simulink model "HybridSystem"  (R2020a)
settings: Solver=FixedStepAuto  StartTime=0  StopTime=1000  FixedStep=0.01  RelTol=1e-3
undefined symbols (not defined in the file): K_I, K_P, n_delay, sac_thresh, switch_thresh, T_lim_low, T_lim_up
libraries: cstblocks x1, simulink x1
settings Model: Creator=Brock  LastModifiedBy=Brock

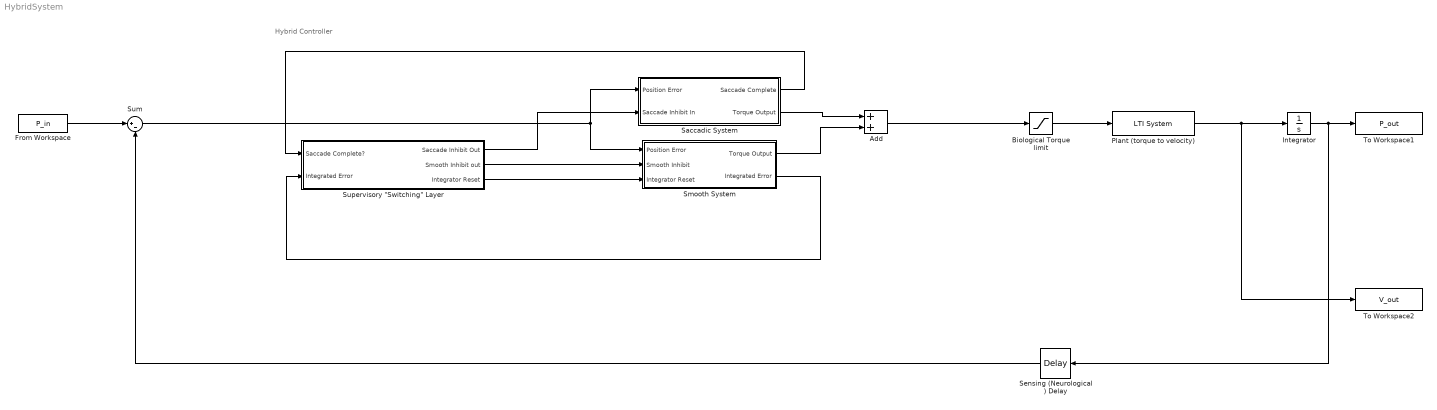
== system HybridSystem ==
  note: Hybrid Controller
  Add : Sum
  Biological Torque limit : Saturate  UpperLimit=T_lim_up  LowerLimit=T_lim_low  LinearizeAsGain=off
  From Workspace : FromWorkspace  VariableName=P_in
  Integrator : Integrator
  Plant (torque to velocity) : cstblocks/LTI System  sys=G_plant  IC=[]
  Saccadic System : Subsystem
  Sensing (Neurological) Delay : TransportDelay  DelayTime=n_delay
  Smooth System : Subsystem
  Sum : Sum  Inputs=|+-
  "Supervisory \"Switching\" Layer" : Subsystem
  To Workspace1 : ToWorkspace  VariableName=P_out  SampleTime=-1
  To Workspace2 : ToWorkspace  VariableName=V_out  SampleTime=-1
  wires:
  From Workspace/1 -> Sum/1
  Plant (torque to velocity)/1 -> Integrator/1, To Workspace2/1
  Integrator/1 -> Sensing (Neurological) Delay/1, To Workspace1/1
  Biological Torque limit/1 -> Plant (torque to velocity)/1
  Sensing (Neurological) Delay/1 -> Sum/2
  Add/1 -> Biological Torque limit/1
  Smooth System/1(Torque Output) -> Add/2
  Saccadic System/2(Torque Output) -> Add/1
  "Supervisory \"Switching\" Layer"/3(Integrator Reset) -> Smooth System/3(Integrator Reset)
  Smooth System/2(Integrated Error) -> "Supervisory \"Switching\" Layer"/2(Integrated Error)
  Sum/1 -> Saccadic System/1(Position Error), Smooth System/1(Position Error)
  Saccadic System/1(Saccade Complete) -> "Supervisory \"Switching\" Layer"/1(Saccade Complete?)
  "Supervisory \"Switching\" Layer"/2(Smooth Inhibit out) -> Smooth System/2(Smooth Inhibit)
  "Supervisory \"Switching\" Layer"/1(Saccade Inhibit Out) -> Saccadic System/2(Saccade Inhibit In)

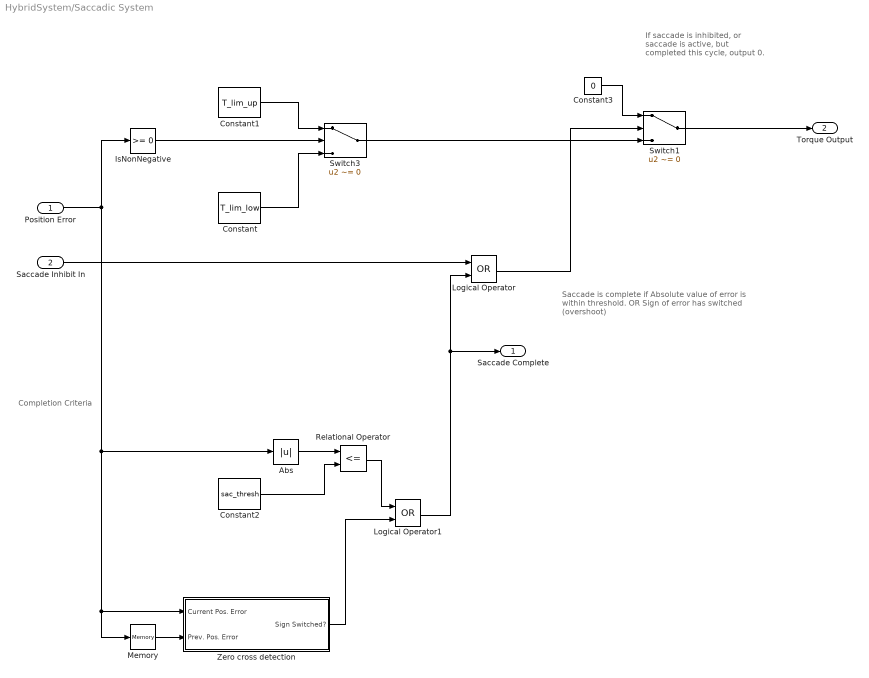
== system HybridSystem/Saccadic System ==
  note: Completion
      | Criteria
  note: If saccade is inhibited, or saccade is active, but completed this cycle, output 0.
  note: Saccade is complete if
      | Absolute value of error is within threshold.
      | OR
      | Sign of error has switched (overshoot)
  Position Error : Inport
  Saccade Inhibit In : Inport  Port=2
  Abs : Abs
  Constant : Constant  Value=T_lim_low
  Constant1 : Constant  Value=T_lim_up
  Constant2 : Constant  Value=sac_thresh
  Constant3 : Constant  Value=0
  IsNonNegative : simulink/Logic and Bit Operations/Compare To Zero  relop=>=  OutDataTypeStr=boolean
  Logical Operator : Logic  Operator=OR  AllPortsSameDT=off  OutDataTypeStr=boolean
  Logical Operator1 : Logic  Operator=OR  AllPortsSameDT=off  OutDataTypeStr=boolean
  Memory : Memory  InheritSampleTime=on
  Relational Operator : RelationalOperator  Operator=<=  OutDataTypeStr=boolean  RndMeth=Simplest
  Switch1 : Switch  Criteria=u2 ~= 0  Threshold=1
  Switch3 : Switch  Criteria=u2 ~= 0
  Zero cross detection : Subsystem
  Saccade Complete : Outport
  Torque Output : Outport  Port=2
  wires:
  Constant2/1 -> Relational Operator/2
  Position Error/1 -> Memory/1, Zero cross detection/1(Current Pos. Error), Abs/1, IsNonNegative/1
  Abs/1 -> Relational Operator/1
  Saccade Inhibit In/1 -> Logical Operator/1
  Switch1/1 -> Torque Output/1
  Constant3/1 -> Switch1/1
  Constant/1 -> Switch3/3
  Constant1/1 -> Switch3/1
  Logical Operator/1 -> Switch1/2
  Switch3/1 -> Switch1/3
  Relational Operator/1 -> Logical Operator1/1
  Logical Operator1/1 -> Logical Operator/2, Saccade Complete/1
  Zero cross detection/1(Sign Switched?) -> Logical Operator1/2
  IsNonNegative/1 -> Switch3/2
  Memory/1 -> Zero cross detection/2(Prev. Pos. Error)

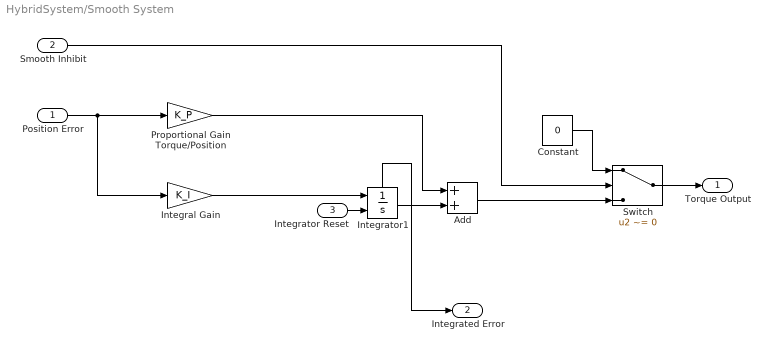
== system HybridSystem/Smooth System ==
  Position Error : Inport
  Smooth Inhibit : Inport  Port=2
  Integrator Reset : Inport  Port=3
  Add : Sum
  Constant : Constant  Value=0
  "Integral Gain " : Gain  Gain=K_I
  Integrator1 : Integrator  ExternalReset=rising  ShowStatePort=on
  Proportional Gain Torque/Position : Gain  Gain=K_P
  Switch : Switch  Criteria=u2 ~= 0
  Torque Output : Outport
  Integrated Error : Outport  Port=2
  wires:
  Proportional Gain Torque/Position/1 -> Add/1
  "Integral Gain "/1 -> Integrator1/1
  Integrator Reset/1 -> Integrator1/2
  Integrator1/1 -> Add/2
  Position Error/1 -> "Integral Gain "/1, Proportional Gain Torque/Position/1
  Switch/1 -> Torque Output/1
  Smooth Inhibit/1 -> Switch/2
  Add/1 -> Switch/3
  Constant/1 -> Switch/1
  Integrator1/State -> Integrated Error/1

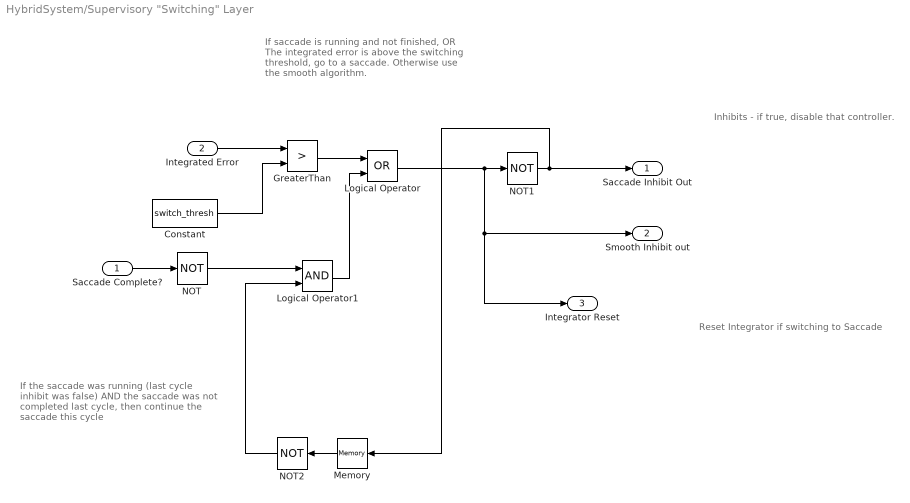
== system HybridSystem/Supervisory "Switching" Layer ==
  note: Inhibits - if true, disable that controller.
  note: If the saccade was running (last cycle inhibit was false)
      | AND the saccade was not completed last cycle, then continue
      | the saccade this cycle
  note: If saccade is running and not finished,
      | OR
      | The integrated error is above the switching threshold, go to a saccade.
      | Otherwise use the smooth algorithm.
  note: Reset Integrator if switching to Saccade
  Saccade Complete? : Inport
  Integrated Error : Inport  Port=2
  Constant : Constant  Value=switch_thresh
  GreaterThan : RelationalOperator  Operator=>  OutDataTypeStr=boolean  RndMeth=Simplest
  Logical Operator : Logic  Operator=OR  AllPortsSameDT=off  OutDataTypeStr=boolean
  Logical Operator1 : Logic  AllPortsSameDT=off  OutDataTypeStr=boolean
  Memory : Memory
  NOT : Logic  Operator=NOT  IconShape=distinctive  AllPortsSameDT=off  OutDataTypeStr=boolean
  NOT1 : Logic  Operator=NOT  IconShape=distinctive  AllPortsSameDT=off  OutDataTypeStr=boolean
  NOT2 : Logic  Operator=NOT  IconShape=distinctive  AllPortsSameDT=off  OutDataTypeStr=boolean
  Saccade Inhibit Out : Outport
  Smooth Inhibit out : Outport  Port=2
  Integrator Reset : Outport  Port=3
  wires:
  Integrated Error/1 -> GreaterThan/1
  Constant/1 -> GreaterThan/2
  Saccade Complete?/1 -> NOT/1
  GreaterThan/1 -> Logical Operator/1
  Logical Operator/1 -> NOT1/1, Smooth Inhibit out/1, Integrator Reset/1
  NOT1/1 -> Memory/1, Saccade Inhibit Out/1
  Logical Operator1/1 -> Logical Operator/2
  NOT/1 -> Logical Operator1/1
  Memory/1 -> NOT2/1
  NOT2/1 -> Logical Operator1/2

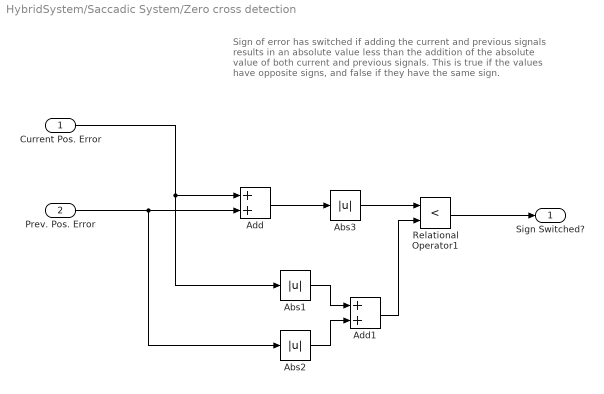
== system HybridSystem/Saccadic System/Zero cross detection ==
  note: Sign of error has switched if adding the current
      | and previous signals results in an absolute value
      | less than the addition of the absolute value of both
      | current and previous signals.
      |
      | This is true if the values have opposite signs, and false
      | if they have the same sign.
  Current Pos. Error : Inport
  Prev. Pos. Error : Inport  Port=2
  Abs1 : Abs
  Abs2 : Abs
  Abs3 : Abs
  Add : Sum
  Add1 : Sum
  Relational Operator1 : RelationalOperator  Operator=<  OutDataTypeStr=boolean  RndMeth=Simplest
  Sign Switched? : Outport
  wires:
  Add/1 -> Abs3/1
  Prev. Pos. Error/1 -> Abs2/1, Add/2
  Current Pos. Error/1 -> Abs1/1, Add/1
  Abs1/1 -> Add1/1
  Add1/1 -> Relational Operator1/2
  Relational Operator1/1 -> Sign Switched?/1
  Abs2/1 -> Add1/2
  Abs3/1 -> Relational Operator1/1
